simulink model "LFC_role_of_R"  (R2014a)
settings: Solver=ode45  StartTime=0.0  StopTime=100  RelTol=1e-3
libraries: cstblocks x3
settings Model: Creator=Divya M  LastModifiedBy=Divya M

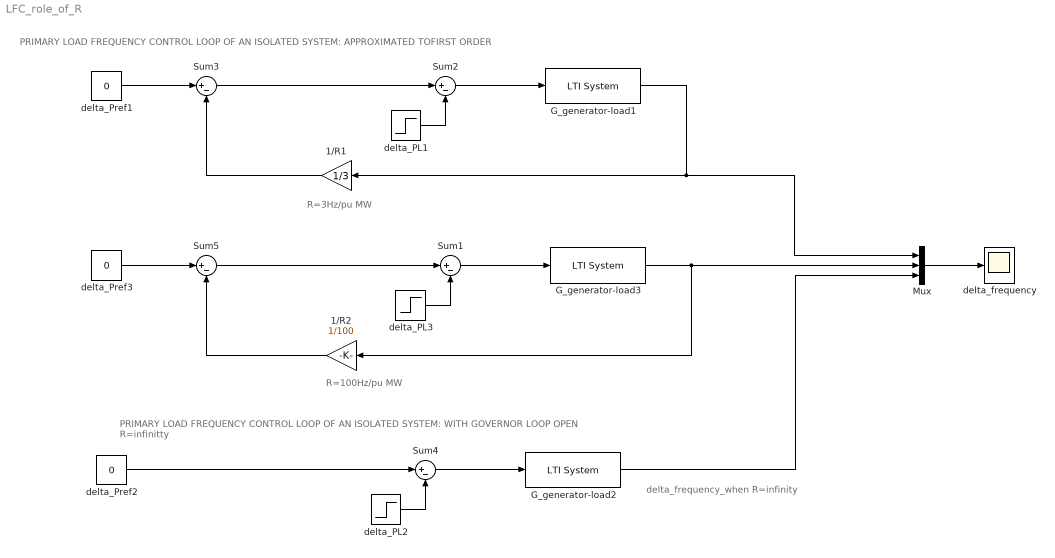
== system LFC_role_of_R ==
  note: R=100Hz/pu MW
  note: R=3Hz/pu MW
  note: PRIMARY LOAD FREQUENCY CONTROL LOOP OF AN ISOLATED SYSTEM: APPROXIMATED TOFIRST ORDER
  note: PRIMARY LOAD FREQUENCY CONTROL LOOP OF AN ISOLATED SYSTEM: WITH GOVERNOR LOOP OPEN R=infinitty
  note: delta_frequency_when R=infinity
  1/R1 : Gain  Gain=1/3
  1/R2 : Gain  Gain=1/100
  G_generator-load1 : cstblocks/LTI System  sys=tf(100,[20 1])  IC=[]
  G_generator-load2 : cstblocks/LTI System  sys=tf(100,[20 1])  IC=[]
  G_generator-load3 : cstblocks/LTI System  sys=tf(100,[20 1])  IC=[]
  Mux : Mux  Inputs=3
  Sum{1..5} (5 alike) : Sum  Inputs=|+-
  delta_PL1 : Step  After=0.01  SampleTime=0
  delta_PL2 : Step  After=0.01  SampleTime=0
  delta_PL3 : Step  After=0.01  SampleTime=0
  delta_Pref1 : Constant  Value=0
  delta_Pref2 : Constant  Value=0
  delta_Pref3 : Constant  Value=0
  delta_frequency : Scope
      settings: YMin=-1  YMax=0.1
  wires:
  delta_Pref1/1 -> Sum3/1
  Sum2/1 -> G_generator-load1/1
  G_generator-load1/1 -> 1/R1/1, Mux/1
  delta_PL1/1 -> Sum2/2
  1/R1/1 -> Sum3/2
  Sum3/1 -> Sum2/1
  Mux/1 -> delta_frequency/1
  Sum4/1 -> G_generator-load2/1
  delta_PL2/1 -> Sum4/2
  delta_Pref2/1 -> Sum4/1
  delta_Pref3/1 -> Sum5/1
  Sum1/1 -> G_generator-load3/1
  G_generator-load3/1 -> Mux/2, 1/R2/1
  delta_PL3/1 -> Sum1/2
  1/R2/1 -> Sum5/2
  Sum5/1 -> Sum1/1
  G_generator-load2/1 -> Mux/3
